simulink model "sdslipxy"  (Simulink 5.0)
settings: Solver=ode45  StartTime=0.0  StopTime=tsim  RelTol=1e-5
values from neighbouring files (symbols this model uses):
  k3 = lqrd(a3,b3,eye(3),diag([1 .01/1000]),Ts)    [tslip1.m]
  Kg = lqr(A,B,Q,R)    [start.m]
  psii = 0.0    (= 0)    [tslip1.m]
  T0 = 44*(u0/10)^2;Vi(1)=u0    [tslip1.m]
  u0 = x(13)    [smis30.m]    (also in tslip1.m = 3.5)
  Vi = XU0(1:7)    [tslip1.m]
  xi = 0    [tslip1.m]
  yi = 1    [tslip1.m]
libraries: simulink x1
settings Model: LastModifiedBy=Admin

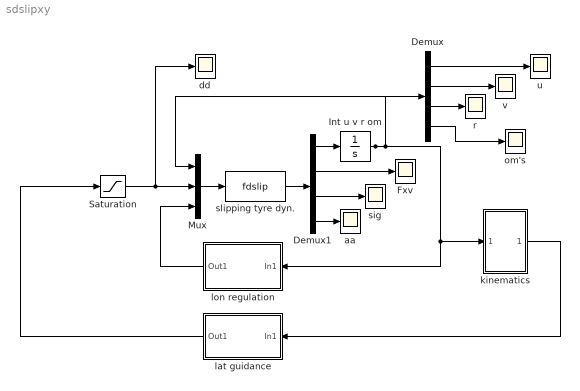
== system sdslipxy ==
  Demux : Demux  Outputs=[1 1 1 4]
  Demux1 : Demux  Outputs=[7 4 4 4]
  Fxv : Scope
      settings: YMin=-25  YMax=150  SaveName=ScopeData5
  Int u v r om : Integrator  InitialCondition=Vi
  Mux : Mux  Inputs=[7 1 1]
  Saturation : Saturate  UpperLimit=0.49  LowerLimit=-0.49
  aa : Scope
      settings: YMin=-0.05  YMax=0.35  SaveName=ScopeData9
  dd : Scope
      settings: YMin=-0.5  YMax=0.5  SaveName=ScopeData3
  kinematics : Subsystem
  lat guidance : Subsystem  Orientation=left
  lon regulation : Subsystem  Orientation=left
  om's : Scope
      settings: YMin=-25  YMax=150  SaveName=ScopeData4
  r : Scope
      settings: YMin=-2  YMax=2
  sig : Scope
      settings: YMin=-0.015  YMax=0.05  SaveName=ScopeData6
  slipping tyre dyn. : MATLABFcn  MATLABFcn=fdslip  OutputDimensions=3+4+3*4
  u : Scope
      settings: YMin=0  YMax=50  SaveName=ScopeData2
  v : Scope
      settings: YMin=-2  YMax=2
  wires:
  Mux/1 -> slipping tyre dyn./1
  slipping tyre dyn./1 -> Demux1/1
  Int u v r om/1 -> Mux/1, Demux/1, kinematics/1(In1), lon regulation/1(In1)
  Demux/1 -> u/1
  Demux/2 -> v/1
  Saturation/1 -> dd/1, Mux/2
  Demux/3 -> r/1
  Demux/4 -> om's/1
  lat guidance/1(Out1) -> Saturation/1
  Demux1/1 -> Int u v r om/1
  Demux1/2 -> Fxv/1
  Demux1/3 -> sig/1
  kinematics/1(Out1) -> lat guidance/1(In1)
  lon regulation/1(Out1) -> Mux/3
  Demux1/4 -> aa/1

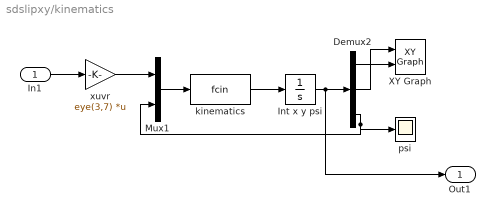
== system sdslipxy/kinematics ==
  In1 : Inport
  Demux2 : Demux  Outputs=3
  Int x y psi : Integrator  InitialCondition=[xi yi psii]
  Mux1 : Mux  Inputs=[3 1]
  XY Graph : simulink/Sinks/XY Graph  xmin=-50  xmax=160  ymin=-50  ymax=160  st=-1
  kinematics : MATLABFcn  MATLABFcn=fcin  OutputDimensions=3
  psi : Scope
      settings: YMin=-2  YMax=2  SaveName=ScopeData7
  xuvr : Gain  Gain=eye(3,7)  Multiplication=Matrix(K*u)  SaturateOnIntegerOverflow=on
  Out1 : Outport
  wires:
  Mux1/1 -> kinematics/1
  kinematics/1 -> Int x y psi/1
  Int x y psi/1 -> Demux2/1, Out1/1
  Demux2/3 -> psi/1, Mux1/2
  Demux2/1 -> XY Graph/2
  Demux2/2 -> XY Graph/1
  xuvr/1 -> Mux1/1
  In1/1 -> xuvr/1

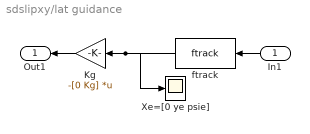
== system sdslipxy/lat guidance ==
  In1 : Inport  Orientation=left
  Kg : Gain  Orientation=left  Gain=-[0 Kg]  Multiplication=Matrix(K*u)  SaturateOnIntegerOverflow=on
  Xe=[0 ye psie] : Scope
      settings: YMin=-1  YMax=3.5  SaveName=ScopeData8
  ftrack : MATLABFcn  Orientation=left  MATLABFcn=ftrack  OutputDimensions=3
  Out1 : Outport  Orientation=left
  wires:
  ftrack/1 -> Xe=[0 ye psie]/1, Kg/1
  Kg/1 -> Out1/1
  In1/1 -> ftrack/1

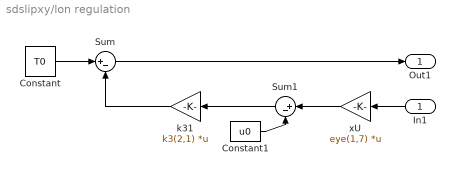
== system sdslipxy/lon regulation ==
  In1 : Inport  Orientation=left
  Constant : Constant  Value=T0
  Constant1 : Constant  Value=u0
  Sum : Sum  Inputs=|+-  SaturateOnIntegerOverflow=on
  Sum1 : Sum  Orientation=left  Inputs=|+-  SaturateOnIntegerOverflow=on
  k31 : Gain  Orientation=left  Gain=k3(2,1)  Multiplication=Matrix(K*u)  SaturateOnIntegerOverflow=on
  xU : Gain  Orientation=left  Gain=eye(1,7)  Multiplication=Matrix(K*u)  SaturateOnIntegerOverflow=on
  Out1 : Outport
  wires:
  Constant/1 -> Sum/1
  k31/1 -> Sum/2
  Sum1/1 -> k31/1
  Constant1/1 -> Sum1/2
  xU/1 -> Sum1/1
  In1/1 -> xU/1
  Sum/1 -> Out1/1
